simulink model "simulink_model"  (R2020b)
settings: Solver=VariableStepAuto  StartTime=0.0  StopTime=90  FixedStep=Ts  RelTol=1e-3
undefined symbols (not defined in the file): DiscIntNeverNeededParam, dist, drv, g, gbox, K, K_e_state, K_I, ms22g, Nr, Nu, Nx, sens, Ts, w_c, wheel
settings Model: Creator=giovanni  LastModifiedBy=giovanni

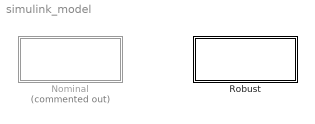
== system simulink_model ==
  Nominal : Subsystem  Commented=on
  Robust : Subsystem

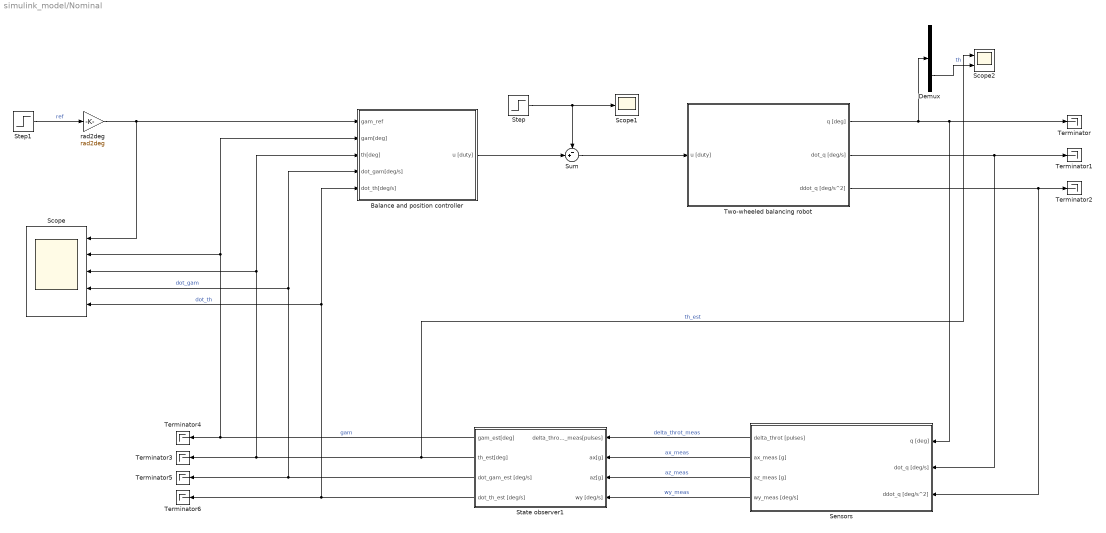
== system simulink_model/Nominal ==
  Balance and position controller : Subsystem
  Demux : Demux  Outputs=2
  Scope : Scope  NumInputPorts=5
  Scope1 : Scope
  Scope2 : Scope  NumInputPorts=2
  "Sensors " : Subsystem
  State observer1 : Subsystem
  Step : Step  Time=10  After=dist  SampleTime=Ts
  Step1 : Step  Time=0  After=step  SampleTime=0
  Sum : Sum  Inputs=-+|
  Terminator{,1..6} (7 alike) : Terminator
  Two-wheeled balancing robot : Subsystem
  rad2deg : Gain  Gain=rad2deg
  wires:
  Two-wheeled balancing robot/2(dot_q [deg/s]) -> "Sensors "/2(dot_q [deg/s]), Terminator1/1
  State observer1/3(dot_gam_est [deg/s]) -> Scope/4, Balance and position controller/4(dot_gam[deg/s]), Terminator5/1  "dot_gam"
  State observer1/4(dot_th_est [deg/s]) -> Scope/5, Balance and position controller/5(dot_th[deg/s]), Terminator6/1  "dot_th"
  Step1/1 -> rad2deg/1  "ref"
  "Sensors "/4(wy_meas [deg/s]) -> State observer1/4(wy [deg/s])  "wy_meas"
  State observer1/2(th_est[deg]) -> Scope2/1, Balance and position controller/3(th[deg]), Scope/3, Terminator3/1  "th_est"
  Two-wheeled balancing robot/3(ddot_q [deg/s^2]) -> "Sensors "/3(ddot_q [deg/s^2]), Terminator2/1
  Sum/1 -> Two-wheeled balancing robot/1(u [duty])
  "Sensors "/1(delta_throt [pulses]) -> State observer1/1(delta_throt_meas[pulses])  "delta_throt_meas"
  State observer1/1(gam_est[deg]) -> Scope/2, Balance and position controller/2(gam[deg]), Terminator4/1  "gam"
  "Sensors "/3(az_meas [g]) -> State observer1/3(az[g])  "az_meas"
  "Sensors "/2(ax_meas [g]) -> State observer1/2(ax[g])  "ax_meas"
  Two-wheeled balancing robot/1(q [deg]) -> Demux/1, "Sensors "/1(q [deg]), Terminator/1
  Balance and position controller/1(u [duty]) -> Sum/2
  Step/1 -> Scope1/1, Sum/1
  rad2deg/1 -> Scope/1, Balance and position controller/1(gam_ref)
  Demux/2 -> Scope2/2  "th"

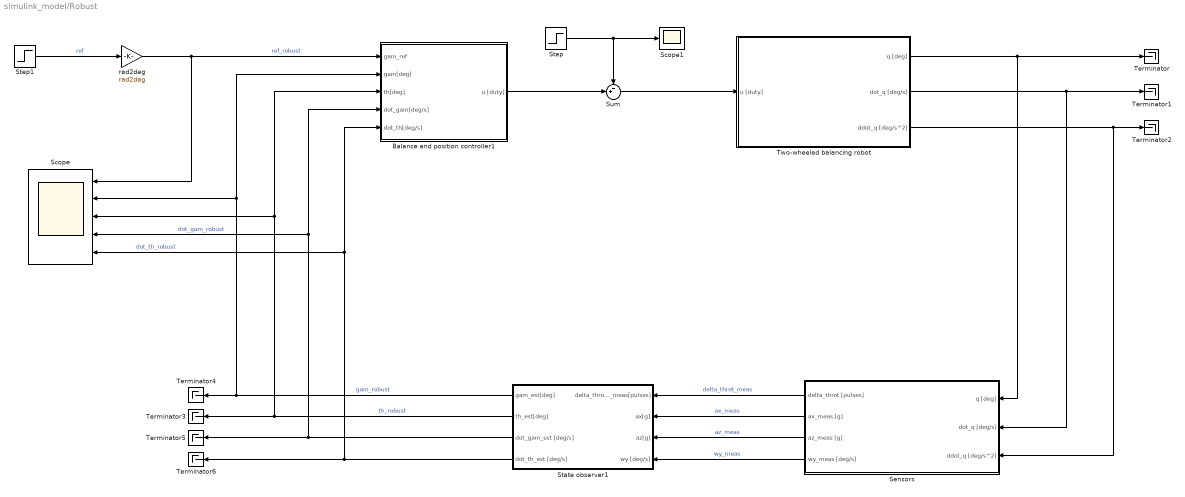
== system simulink_model/Robust ==
  Balance and position controller1 : Subsystem
  Scope : Scope  NumInputPorts=5
  Scope1 : Scope
  "Sensors " : Subsystem
  State observer1 : Subsystem
  Step : Step  Time=10  After=dist  SampleTime=Ts
  Step1 : Step  Time=0  After=step  SampleTime=0
  Sum : Sum  Inputs=-+|
  Terminator{,1..6} (7 alike) : Terminator
  Two-wheeled balancing robot : Subsystem
  rad2deg : Gain  Gain=rad2deg
  wires:
  Two-wheeled balancing robot/2(dot_q [deg/s]) -> "Sensors "/2(dot_q [deg/s]), Terminator1/1
  State observer1/3(dot_gam_est [deg/s]) -> Balance and position controller1/4(dot_gam[deg/s]), Scope/4, Terminator5/1  "dot_gam_robust"
  State observer1/4(dot_th_est [deg/s]) -> Balance and position controller1/5(dot_th[deg/s]), Scope/5, Terminator6/1  "dot_th_robust"
  Step1/1 -> rad2deg/1  "ref"
  "Sensors "/4(wy_meas [deg/s]) -> State observer1/4(wy [deg/s])  "wy_meas"
  State observer1/2(th_est[deg]) -> Balance and position controller1/3(th[deg]), Scope/3, Terminator3/1  "th_robust"
  Two-wheeled balancing robot/3(ddot_q [deg/s^2]) -> "Sensors "/3(ddot_q [deg/s^2]), Terminator2/1
  Sum/1 -> Two-wheeled balancing robot/1(u [duty])
  "Sensors "/1(delta_throt [pulses]) -> State observer1/1(delta_throt_meas[pulses])  "delta_throt_meas"
  State observer1/1(gam_est[deg]) -> Balance and position controller1/2(gam[deg]), Scope/2, Terminator4/1  "gam_robust"
  "Sensors "/3(az_meas [g]) -> State observer1/3(az[g])  "az_meas"
  "Sensors "/2(ax_meas [g]) -> State observer1/2(ax[g])  "ax_meas"
  Two-wheeled balancing robot/1(q [deg]) -> "Sensors "/1(q [deg]), Terminator/1
  Balance and position controller1/1(u [duty]) -> Sum/2
  Step/1 -> Scope1/1, Sum/1
  rad2deg/1 -> Balance and position controller1/1(gam_ref), Scope/1  "ref_robust"

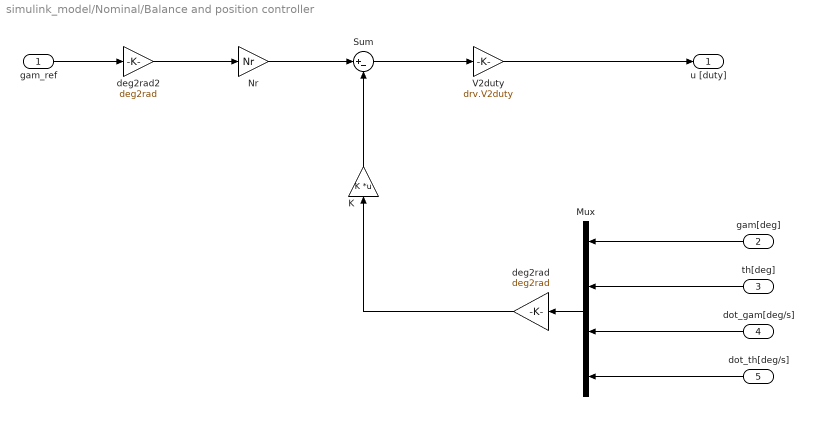
== system simulink_model/Nominal/Balance and position controller ==
  gam_ref : Inport
  gam[deg] : Inport  Port=2
  th[deg] : Inport  Port=3
  dot_gam[deg/s] : Inport  Port=4
  dot_th[deg/s] : Inport  Port=5
  K : Gain  Gain=K  Multiplication=Matrix(K*u)
  Mux : Mux
  Nr : Gain  Gain=Nr
  Sum : Sum  Inputs=|+-
  V2duty : Gain  Gain=drv.V2duty
  deg2rad : Gain  Gain=deg2rad
  deg2rad2 : Gain  Gain=deg2rad
  u [duty] : Outport
  wires:
  Nr/1 -> Sum/1
  gam_ref/1 -> deg2rad2/1
  deg2rad2/1 -> Nr/1
  Sum/1 -> V2duty/1
  V2duty/1 -> u [duty]/1
  deg2rad/1 -> K/1
  K/1 -> Sum/2
  Mux/1 -> deg2rad/1
  gam[deg]/1 -> Mux/1
  dot_th[deg/s]/1 -> Mux/4
  th[deg]/1 -> Mux/2
  dot_gam[deg/s]/1 -> Mux/3

== system simulink_model/Nominal/Sensors  ==
  q [deg] : Inport
  dot_q [deg/s] : Inport  Port=2
  ddot_q [deg/s^2] : Inport  Port=3
  Accelerometer : Subsystem
  Encoder : Subsystem
  Gyroscope : Subsystem
  delta_throt [pulses] : Outport
  ax_meas [g] : Outport  Port=2
  az_meas [g] : Outport  Port=3
  wy_meas [deg/s] : Outport  Port=4
  wires:
  ddot_q [deg/s^2]/1 -> Accelerometer/3(ddot_q [deg/s^2])
  dot_q [deg/s]/1 -> Gyroscope/1(dot_q [deg/s]), Accelerometer/2(dot_q [deg/s])
  q [deg]/1 -> Encoder/1(q [deg]), Accelerometer/1(q [deg])
  Accelerometer/1(ax [g]) -> ax_meas [g]/1
  Accelerometer/2(az [g]) -> az_meas [g]/1
  Gyroscope/1(wy [deg/s]) -> wy_meas [deg/s]/1
  Encoder/1(delta_throt [pulses]) -> delta_throt [pulses]/1

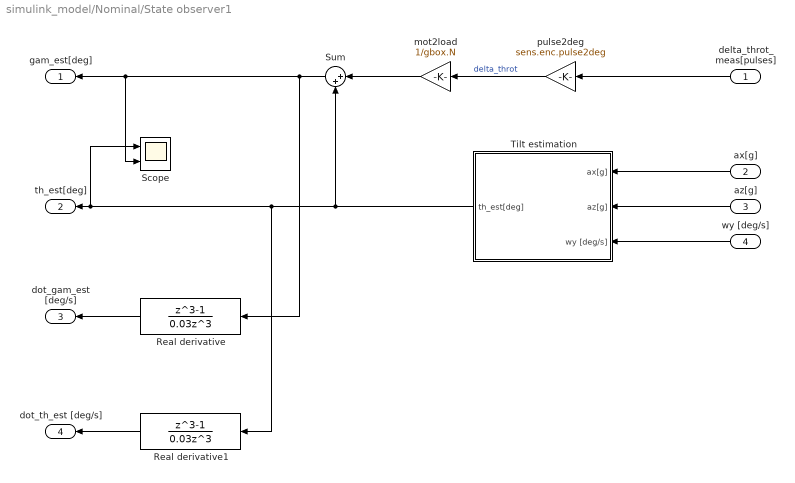
== system simulink_model/Nominal/State observer1 ==
  delta_throt_meas[pulses] : Inport
  ax[g] : Inport  Port=2
  az[g] : Inport  Port=3
  wy [deg/s] : Inport  Port=4
  Real derivative : DiscreteTransferFcn  Numerator=[1 0 0 -1]  Denominator=[0.03 0 0 0]
  Real derivative1 : DiscreteTransferFcn  Numerator=[1 0 0 -1]  Denominator=[0.03 0 0 0]
  Scope : Scope  NumInputPorts=2
  Sum : Sum  Inputs=|++
  "Tilt estimation " : Subsystem
  mot2load : Gain  Gain=1/gbox.N
  pulse2deg : Gain  Gain=sens.enc.pulse2deg
  gam_est[deg] : Outport
  th_est[deg] : Outport  Port=2
  dot_gam_est [deg/s] : Outport  Port=3
  dot_th_est [deg/s] : Outport  Port=4
  wires:
  wy [deg/s]/1 -> "Tilt estimation "/3(wy [deg/s])
  ax[g]/1 -> "Tilt estimation "/1(ax[g])
  az[g]/1 -> "Tilt estimation "/2(az[g])
  delta_throt_meas[pulses]/1 -> pulse2deg/1
  pulse2deg/1 -> mot2load/1  "delta_throt"
  mot2load/1 -> Sum/1
  "Tilt estimation "/1(th_est[deg]) -> Scope/1, th_est[deg]/1, Real derivative1/1, Sum/2
  Sum/1 -> Scope/2, gam_est[deg]/1, Real derivative/1
  Real derivative/1 -> dot_gam_est [deg/s]/1
  Real derivative1/1 -> dot_th_est [deg/s]/1

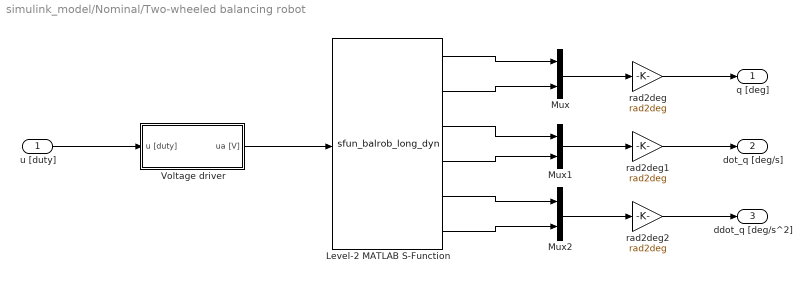
== system simulink_model/Nominal/Two-wheeled balancing robot ==
  u [duty] : Inport
  Level-2 MATLAB S-Function : M-S-Function  FunctionName=sfun_balrob_long_dyn  Parameters=x0, body, mot, gbox, wheel
  Mux : Mux  Inputs=2
  Mux1 : Mux  Inputs=2
  Mux2 : Mux  Inputs=2
  Voltage driver : Subsystem
  rad2deg : Gain  Gain=rad2deg
  rad2deg1 : Gain  Gain=rad2deg
  rad2deg2 : Gain  Gain=rad2deg
  q [deg] : Outport
  dot_q [deg/s] : Outport  Port=2
  ddot_q [deg/s^2] : Outport  Port=3
  wires:
  Level-2 MATLAB S-Function/2 -> Mux/2
  rad2deg2/1 -> ddot_q [deg/s^2]/1
  Level-2 MATLAB S-Function/1 -> Mux/1
  Mux/1 -> rad2deg/1
  rad2deg/1 -> q [deg]/1
  Level-2 MATLAB S-Function/5 -> Mux2/1
  Mux2/1 -> rad2deg2/1
  Level-2 MATLAB S-Function/4 -> Mux1/2
  Mux1/1 -> rad2deg1/1
  Level-2 MATLAB S-Function/3 -> Mux1/1
  rad2deg1/1 -> dot_q [deg/s]/1
  Level-2 MATLAB S-Function/6 -> Mux2/2
  Voltage driver/1(ua [V]) -> Level-2 MATLAB S-Function/1
  u [duty]/1 -> Voltage driver/1(u [duty])

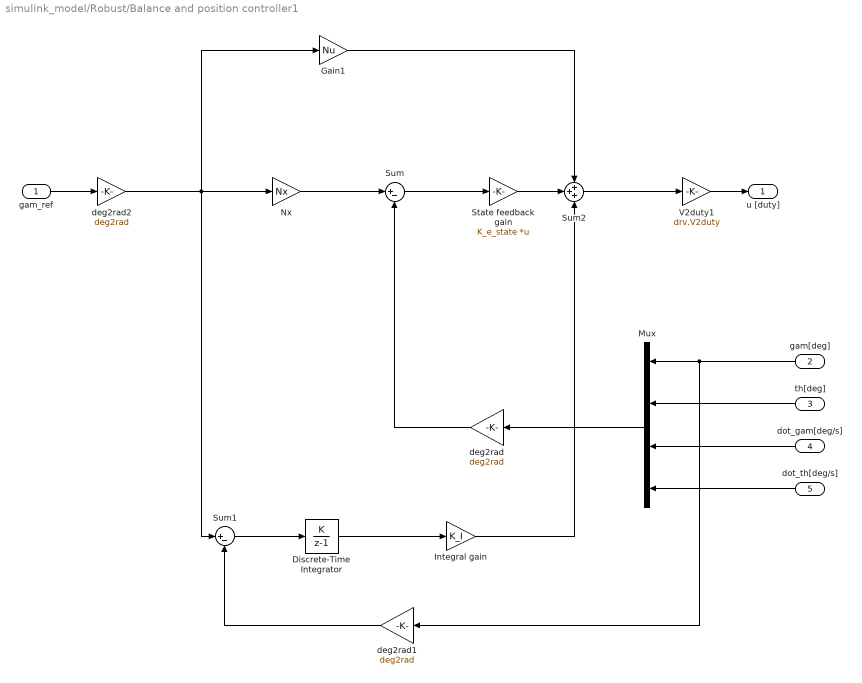
== system simulink_model/Robust/Balance and position controller1 ==
  gam_ref : Inport
  gam[deg] : Inport  Port=2
  th[deg] : Inport  Port=3
  dot_gam[deg/s] : Inport  Port=4
  dot_th[deg/s] : Inport  Port=5
  Discrete-Time Integrator : DiscreteIntegrator  IntegratorMethod=Accumulation: Forward Euler  SampleTime=-1  ICPrevOutput=DiscIntNeverNeededParam  ICPrevScaledInput=DiscIntNeverNeededParam
  Gain1 : Gain  Gain=Nu
  Integral gain : Gain  Gain=K_I
  Mux : Mux
  Nx : Gain  Gain=Nx
  State feedback gain : Gain  Gain=K_e_state  Multiplication=Matrix(K*u)
  Sum : Sum  Inputs=|+-
  Sum1 : Sum  Inputs=|+-
  Sum2 : Sum  Inputs=+++
  V2duty1 : Gain  Gain=drv.V2duty
  deg2rad : Gain  Gain=deg2rad
  deg2rad1 : Gain  Gain=deg2rad
  deg2rad2 : Gain  Gain=deg2rad
  u [duty] : Outport
  wires:
  Nx/1 -> Sum/1
  gam_ref/1 -> deg2rad2/1
  deg2rad2/1 -> Gain1/1, Sum1/1, Nx/1
  V2duty1/1 -> u [duty]/1
  deg2rad/1 -> Sum/2
  Mux/1 -> deg2rad/1
  dot_th[deg/s]/1 -> Mux/4
  th[deg]/1 -> Mux/2
  dot_gam[deg/s]/1 -> Mux/3
  gam[deg]/1 -> deg2rad1/1, Mux/1
  deg2rad1/1 -> Sum1/2
  Sum1/1 -> Discrete-Time Integrator/1
  Discrete-Time Integrator/1 -> Integral gain/1
  Sum/1 -> State feedback gain/1
  Integral gain/1 -> Sum2/3
  Gain1/1 -> Sum2/1
  State feedback gain/1 -> Sum2/2
  Sum2/1 -> V2duty1/1

== system simulink_model/Robust/Sensors  ==
  q [deg] : Inport
  dot_q [deg/s] : Inport  Port=2
  ddot_q [deg/s^2] : Inport  Port=3
  Accelerometer : Subsystem
  Encoder : Subsystem
  Gyroscope : Subsystem
  delta_throt [pulses] : Outport
  ax_meas [g] : Outport  Port=2
  az_meas [g] : Outport  Port=3
  wy_meas [deg/s] : Outport  Port=4
  wires:
  ddot_q [deg/s^2]/1 -> Accelerometer/3(ddot_q [deg/s^2])
  dot_q [deg/s]/1 -> Gyroscope/1(dot_q [deg/s]), Accelerometer/2(dot_q [deg/s])
  q [deg]/1 -> Encoder/1(q [deg]), Accelerometer/1(q [deg])
  Accelerometer/1(ax [g]) -> ax_meas [g]/1
  Accelerometer/2(az [g]) -> az_meas [g]/1
  Gyroscope/1(wy [deg/s]) -> wy_meas [deg/s]/1
  Encoder/1(delta_throt [pulses]) -> delta_throt [pulses]/1

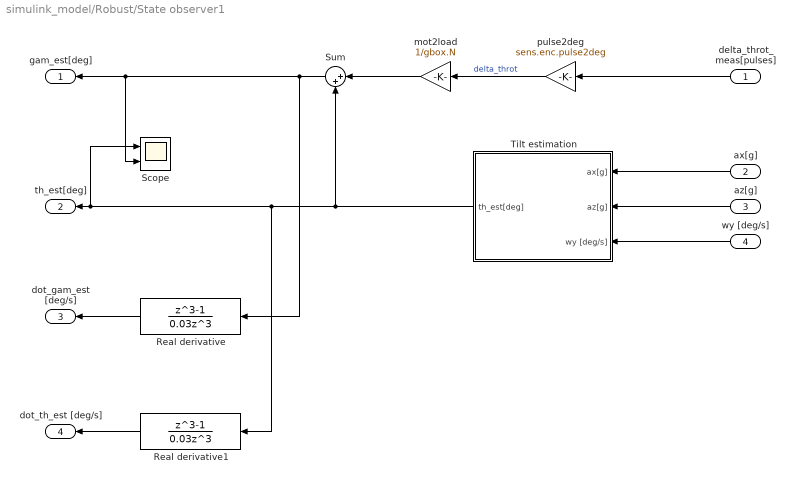
== system simulink_model/Robust/State observer1 ==
  delta_throt_meas[pulses] : Inport
  ax[g] : Inport  Port=2
  az[g] : Inport  Port=3
  wy [deg/s] : Inport  Port=4
  Real derivative : DiscreteTransferFcn  Numerator=[1 0 0 -1]  Denominator=[0.03 0 0 0]
  Real derivative1 : DiscreteTransferFcn  Numerator=[1 0 0 -1]  Denominator=[0.03 0 0 0]
  Scope : Scope  NumInputPorts=2
  Sum : Sum  Inputs=|++
  "Tilt estimation " : Subsystem
  mot2load : Gain  Gain=1/gbox.N
  pulse2deg : Gain  Gain=sens.enc.pulse2deg
  gam_est[deg] : Outport
  th_est[deg] : Outport  Port=2
  dot_gam_est [deg/s] : Outport  Port=3
  dot_th_est [deg/s] : Outport  Port=4
  wires:
  wy [deg/s]/1 -> "Tilt estimation "/3(wy [deg/s])
  ax[g]/1 -> "Tilt estimation "/1(ax[g])
  az[g]/1 -> "Tilt estimation "/2(az[g])
  delta_throt_meas[pulses]/1 -> pulse2deg/1
  pulse2deg/1 -> mot2load/1  "delta_throt"
  mot2load/1 -> Sum/1
  "Tilt estimation "/1(th_est[deg]) -> Scope/1, th_est[deg]/1, Real derivative1/1, Sum/2
  Sum/1 -> Scope/2, gam_est[deg]/1, Real derivative/1
  Real derivative/1 -> dot_gam_est [deg/s]/1
  Real derivative1/1 -> dot_th_est [deg/s]/1

== system simulink_model/Robust/Two-wheeled balancing robot ==
  u [duty] : Inport
  Level-2 MATLAB S-Function : M-S-Function  FunctionName=sfun_balrob_long_dyn  Parameters=x0, body, mot, gbox, wheel
  Mux : Mux  Inputs=2
  Mux1 : Mux  Inputs=2
  Mux2 : Mux  Inputs=2
  Voltage driver : Subsystem
  rad2deg : Gain  Gain=rad2deg
  rad2deg1 : Gain  Gain=rad2deg
  rad2deg2 : Gain  Gain=rad2deg
  q [deg] : Outport
  dot_q [deg/s] : Outport  Port=2
  ddot_q [deg/s^2] : Outport  Port=3
  wires:
  Level-2 MATLAB S-Function/2 -> Mux/2
  rad2deg2/1 -> ddot_q [deg/s^2]/1
  Level-2 MATLAB S-Function/1 -> Mux/1
  Mux/1 -> rad2deg/1
  rad2deg/1 -> q [deg]/1
  Level-2 MATLAB S-Function/5 -> Mux2/1
  Mux2/1 -> rad2deg2/1
  Level-2 MATLAB S-Function/4 -> Mux1/2
  Mux1/1 -> rad2deg1/1
  Level-2 MATLAB S-Function/3 -> Mux1/1
  rad2deg1/1 -> dot_q [deg/s]/1
  Level-2 MATLAB S-Function/6 -> Mux2/2
  Voltage driver/1(ua [V]) -> Level-2 MATLAB S-Function/1
  u [duty]/1 -> Voltage driver/1(u [duty])

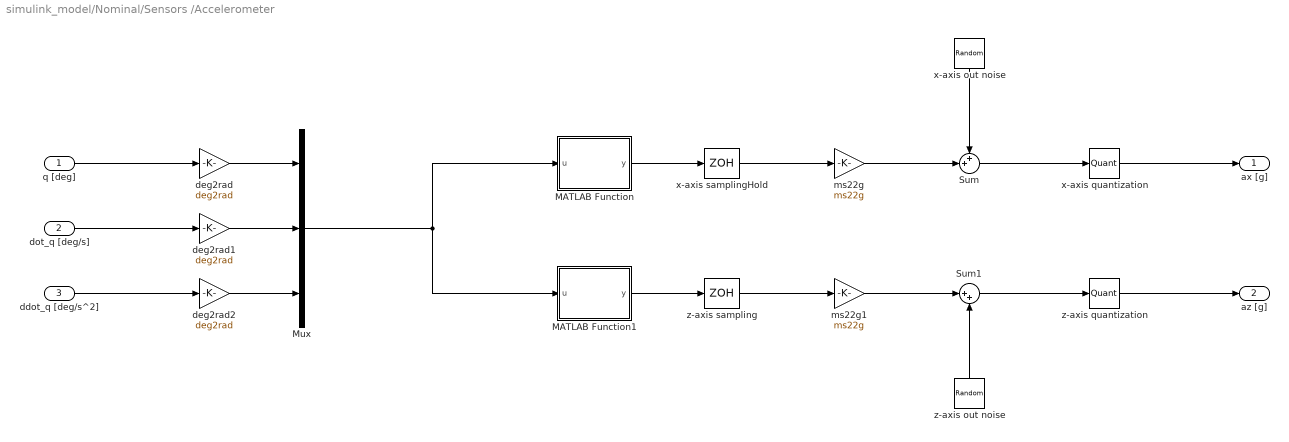
== system simulink_model/Nominal/Sensors /Accelerometer ==
  q [deg] : Inport
  dot_q [deg/s] : Inport  Port=2
  ddot_q [deg/s^2] : Inport  Port=3
  MATLAB Function : MATLAB Function  TreatAsAtomicUnit=on
  MATLAB Function1 : MATLAB Function  TreatAsAtomicUnit=on
  Mux : Mux  Inputs=3
  Sum : Sum  Inputs=++|
  Sum1 : Sum  Inputs=|++
  deg2rad : Gain  Gain=deg2rad
  deg2rad1 : Gain  Gain=deg2rad
  deg2rad2 : Gain  Gain=deg2rad
  ms22g : Gain  Gain=ms22g
  ms22g1 : Gain  Gain=ms22g
  "x-axis out noise " : RandomNumber  Variance=sens.mpu.acc.noisevar  SampleTime=Ts
  x-axis quantization : Quantizer  QuantizationInterval=sens.mpu.acc.LSB2g
  x-axis samplingHold : ZeroOrderHold  SampleTime=Ts
  "z-axis out noise " : RandomNumber  Variance=sens.mpu.acc.noisevar  SampleTime=Ts
  z-axis quantization : Quantizer  QuantizationInterval=sens.mpu.acc.LSB2g
  z-axis sampling : ZeroOrderHold  SampleTime=Ts
  ax [g] : Outport
  az [g] : Outport  Port=2
  wires:
  q [deg]/1 -> deg2rad/1
  dot_q [deg/s]/1 -> deg2rad1/1
  ddot_q [deg/s^2]/1 -> deg2rad2/1
  deg2rad/1 -> Mux/1
  deg2rad1/1 -> Mux/2
  deg2rad2/1 -> Mux/3
  Mux/1 -> MATLAB Function1/1(u), MATLAB Function/1(u)
  MATLAB Function1/1(y) -> z-axis sampling/1
  MATLAB Function/1(y) -> x-axis samplingHold/1
  x-axis samplingHold/1 -> ms22g/1
  z-axis sampling/1 -> ms22g1/1
  ms22g/1 -> Sum/2
  "x-axis out noise "/1 -> Sum/1
  ms22g1/1 -> Sum1/1
  "z-axis out noise "/1 -> Sum1/2
  Sum1/1 -> z-axis quantization/1
  Sum/1 -> x-axis quantization/1
  x-axis quantization/1 -> ax [g]/1
  z-axis quantization/1 -> az [g]/1

== system simulink_model/Nominal/Sensors /Encoder ==
  q [deg] : Inport
  Demux1 : Demux  Outputs=2
  Encoder quantization : Quantizer  QuantizationInterval=sens.enc.pulse2deg
  Encoder sampling : ZeroOrderHold  SampleTime=Ts
  Sum : Sum  Inputs=+-
  deg2pulse : Gain  Gain=sens.enc.deg2pulse
  load2mot : Gain  Gain=gbox.N
  delta_throt [pulses] : Outport
  wires:
  q [deg]/1 -> Demux1/1
  Demux1/1 -> Sum/1
  Demux1/2 -> Sum/2
  Sum/1 -> load2mot/1
  load2mot/1 -> Encoder sampling/1  "delta_throt"
  Encoder sampling/1 -> Encoder quantization/1
  Encoder quantization/1 -> deg2pulse/1
  deg2pulse/1 -> delta_throt [pulses]/1

== system simulink_model/Nominal/Sensors /Gyroscope ==
  dot_q [deg/s] : Inport
  Quantizer : Quantizer  QuantizationInterval=sens.mpu.gyro.LSB2degs
  Random Number : RandomNumber  Variance=sens.mpu.gyro.noisevar  SampleTime=Ts
  Selector : Selector  InputPortWidth=2  IndexOptions=Index vector (dialog)  Indices=[2]  OutputSizes=1
  Sum : Sum  Inputs=++|
  y-axis sampling : ZeroOrderHold  SampleTime=Ts
  wy [deg/s] : Outport
  wires:
  dot_q [deg/s]/1 -> Selector/1
  Selector/1 -> y-axis sampling/1
  y-axis sampling/1 -> Sum/2
  Sum/1 -> Quantizer/1
  Quantizer/1 -> wy [deg/s]/1
  Random Number/1 -> Sum/1

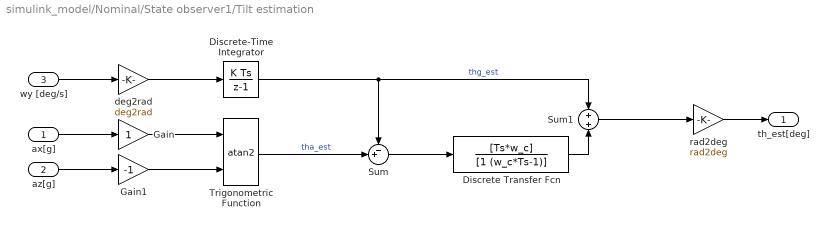
== system simulink_model/Nominal/State observer1/Tilt estimation  ==
  ax[g] : Inport
  az[g] : Inport  Port=2
  wy [deg/s] : Inport  Port=3
  Discrete Transfer Fcn : DiscreteTransferFcn  Numerator=[Ts*w_c]  Denominator=[1 (w_c*Ts-1)]  SampleTime=Ts
  Discrete-Time Integrator : DiscreteIntegrator  SampleTime=Ts  ICPrevOutput=DiscIntNeverNeededParam  ICPrevScaledInput=DiscIntNeverNeededParam
  Gain : Gain
  Gain1 : Gain  Gain=-1
  Sum : Sum  Inputs=-+|
  Sum1 : Sum  Inputs=+|+
  Trigonometric Function : Trigonometry  Operator=atan2
  deg2rad : Gain  Gain=deg2rad
  rad2deg : Gain  Gain=rad2deg
  th_est[deg] : Outport
  wires:
  wy [deg/s]/1 -> deg2rad/1
  az[g]/1 -> Gain1/1
  ax[g]/1 -> Gain/1
  deg2rad/1 -> Discrete-Time Integrator/1
  Gain/1 -> Trigonometric Function/1
  Gain1/1 -> Trigonometric Function/2
  Trigonometric Function/1 -> Sum/2  "tha_est"
  Discrete-Time Integrator/1 -> Sum1/1, Sum/1  "thg_est"
  Sum/1 -> Discrete Transfer Fcn/1
  Discrete Transfer Fcn/1 -> Sum1/2
  Sum1/1 -> rad2deg/1
  rad2deg/1 -> th_est[deg]/1

== system simulink_model/Nominal/Two-wheeled balancing robot/Voltage driver ==
  u [duty] : Inport
  Duty saturation : Saturate  UpperLimit=drv.dutymax  LowerLimit=-drv.dutymax
  Rounding Function : Rounding  Operator=fix
  Zero-Order Hold : ZeroOrderHold  SampleTime=Ts
  duty2V : Gain  Gain=drv.duty2V
  voltage saturation : Saturate  UpperLimit=drv.Vbus  LowerLimit=-drv.Vbus
  ua [V] : Outport
  wires:
  Zero-Order Hold/1 -> ua [V]/1
  duty2V/1 -> voltage saturation/1
  Rounding Function/1 -> duty2V/1
  Duty saturation/1 -> Rounding Function/1
  u [duty]/1 -> Duty saturation/1
  voltage saturation/1 -> Zero-Order Hold/1

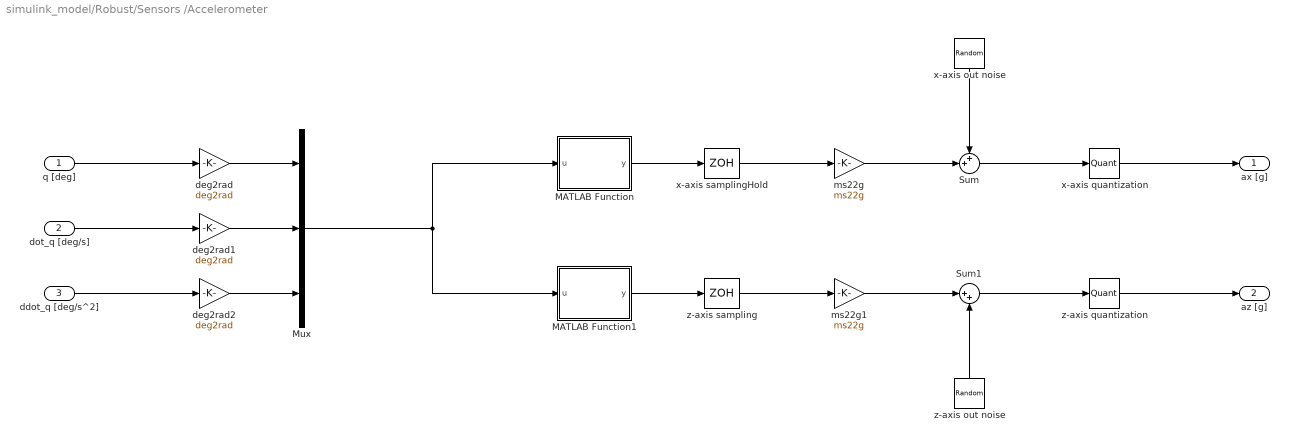
== system simulink_model/Robust/Sensors /Accelerometer ==
  q [deg] : Inport
  dot_q [deg/s] : Inport  Port=2
  ddot_q [deg/s^2] : Inport  Port=3
  MATLAB Function : MATLAB Function  TreatAsAtomicUnit=on
  MATLAB Function1 : MATLAB Function  TreatAsAtomicUnit=on
  Mux : Mux  Inputs=3
  Sum : Sum  Inputs=++|
  Sum1 : Sum  Inputs=|++
  deg2rad : Gain  Gain=deg2rad
  deg2rad1 : Gain  Gain=deg2rad
  deg2rad2 : Gain  Gain=deg2rad
  ms22g : Gain  Gain=ms22g
  ms22g1 : Gain  Gain=ms22g
  "x-axis out noise " : RandomNumber  Variance=sens.mpu.acc.noisevar  SampleTime=Ts
  x-axis quantization : Quantizer  QuantizationInterval=sens.mpu.acc.LSB2g
  x-axis samplingHold : ZeroOrderHold  SampleTime=Ts
  "z-axis out noise " : RandomNumber  Variance=sens.mpu.acc.noisevar  SampleTime=Ts
  z-axis quantization : Quantizer  QuantizationInterval=sens.mpu.acc.LSB2g
  z-axis sampling : ZeroOrderHold  SampleTime=Ts
  ax [g] : Outport
  az [g] : Outport  Port=2
  wires:
  q [deg]/1 -> deg2rad/1
  dot_q [deg/s]/1 -> deg2rad1/1
  ddot_q [deg/s^2]/1 -> deg2rad2/1
  deg2rad/1 -> Mux/1
  deg2rad1/1 -> Mux/2
  deg2rad2/1 -> Mux/3
  Mux/1 -> MATLAB Function1/1(u), MATLAB Function/1(u)
  MATLAB Function1/1(y) -> z-axis sampling/1
  MATLAB Function/1(y) -> x-axis samplingHold/1
  x-axis samplingHold/1 -> ms22g/1
  z-axis sampling/1 -> ms22g1/1
  ms22g/1 -> Sum/2
  "x-axis out noise "/1 -> Sum/1
  ms22g1/1 -> Sum1/1
  "z-axis out noise "/1 -> Sum1/2
  Sum1/1 -> z-axis quantization/1
  Sum/1 -> x-axis quantization/1
  x-axis quantization/1 -> ax [g]/1
  z-axis quantization/1 -> az [g]/1

== system simulink_model/Robust/Sensors /Encoder ==
  q [deg] : Inport
  Demux1 : Demux  Outputs=2
  Encoder quantization : Quantizer  QuantizationInterval=sens.enc.pulse2deg
  Encoder sampling : ZeroOrderHold  SampleTime=Ts
  Sum : Sum  Inputs=+-
  deg2pulse : Gain  Gain=sens.enc.deg2pulse
  load2mot : Gain  Gain=gbox.N
  delta_throt [pulses] : Outport
  wires:
  q [deg]/1 -> Demux1/1
  Demux1/1 -> Sum/1
  Demux1/2 -> Sum/2
  Sum/1 -> load2mot/1
  load2mot/1 -> Encoder sampling/1  "delta_throt"
  Encoder sampling/1 -> Encoder quantization/1
  Encoder quantization/1 -> deg2pulse/1
  deg2pulse/1 -> delta_throt [pulses]/1

== system simulink_model/Robust/Sensors /Gyroscope ==
  dot_q [deg/s] : Inport
  Quantizer : Quantizer  QuantizationInterval=sens.mpu.gyro.LSB2degs
  Random Number : RandomNumber  Variance=sens.mpu.gyro.noisevar  SampleTime=Ts
  Selector : Selector  InputPortWidth=2  IndexOptions=Index vector (dialog)  Indices=[2]  OutputSizes=1
  Sum : Sum  Inputs=++|
  y-axis sampling : ZeroOrderHold  SampleTime=Ts
  wy [deg/s] : Outport
  wires:
  dot_q [deg/s]/1 -> Selector/1
  Selector/1 -> y-axis sampling/1
  y-axis sampling/1 -> Sum/2
  Sum/1 -> Quantizer/1
  Quantizer/1 -> wy [deg/s]/1
  Random Number/1 -> Sum/1

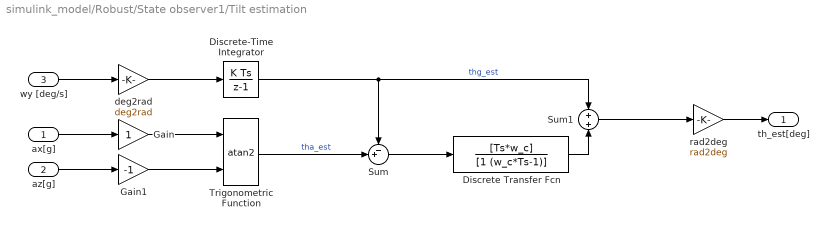
== system simulink_model/Robust/State observer1/Tilt estimation  ==
  ax[g] : Inport
  az[g] : Inport  Port=2
  wy [deg/s] : Inport  Port=3
  Discrete Transfer Fcn : DiscreteTransferFcn  Numerator=[Ts*w_c]  Denominator=[1 (w_c*Ts-1)]  SampleTime=Ts
  Discrete-Time Integrator : DiscreteIntegrator  SampleTime=Ts  ICPrevOutput=DiscIntNeverNeededParam  ICPrevScaledInput=DiscIntNeverNeededParam
  Gain : Gain
  Gain1 : Gain  Gain=-1
  Sum : Sum  Inputs=-+|
  Sum1 : Sum  Inputs=+|+
  Trigonometric Function : Trigonometry  Operator=atan2
  deg2rad : Gain  Gain=deg2rad
  rad2deg : Gain  Gain=rad2deg
  th_est[deg] : Outport
  wires:
  wy [deg/s]/1 -> deg2rad/1
  az[g]/1 -> Gain1/1
  ax[g]/1 -> Gain/1
  deg2rad/1 -> Discrete-Time Integrator/1
  Gain/1 -> Trigonometric Function/1
  Gain1/1 -> Trigonometric Function/2
  Trigonometric Function/1 -> Sum/2  "tha_est"
  Discrete-Time Integrator/1 -> Sum1/1, Sum/1  "thg_est"
  Sum/1 -> Discrete Transfer Fcn/1
  Discrete Transfer Fcn/1 -> Sum1/2
  Sum1/1 -> rad2deg/1
  rad2deg/1 -> th_est[deg]/1

== system simulink_model/Robust/Two-wheeled balancing robot/Voltage driver ==
  u [duty] : Inport
  Duty saturation : Saturate  UpperLimit=drv.dutymax  LowerLimit=-drv.dutymax
  Rounding Function : Rounding  Operator=fix
  Zero-Order Hold : ZeroOrderHold  SampleTime=Ts
  duty2V : Gain  Gain=drv.duty2V
  voltage saturation : Saturate  UpperLimit=drv.Vbus  LowerLimit=-drv.Vbus
  ua [V] : Outport
  wires:
  Zero-Order Hold/1 -> ua [V]/1
  duty2V/1 -> voltage saturation/1
  Rounding Function/1 -> duty2V/1
  Duty saturation/1 -> Rounding Function/1
  u [duty]/1 -> Duty saturation/1
  voltage saturation/1 -> Zero-Order Hold/1

== matlab function simulink_model/Robust/Sensors /Accelerometer/MATLAB Function ==
  data: u input; y output; wheel parameter; sens parameter; g parameter
function y = acc_out_x(u, wheel, sens, g)

y = wheel.r*u(5)*cos(u(2)) + sens.mpu.zb*u(6) + g*sin(u(2));

== matlab function simulink_model/Robust/Sensors /Accelerometer/MATLAB Function1 ==
  data: u input; y output; wheel parameter; sens parameter; g parameter
function y = acc_out_z(u, wheel, sens, g)

y = wheel.r*u(5)*sin(u(2)) - sens.mpu.zb*u(4)^2 - g*cos(u(2));

== matlab function simulink_model/Nominal/Sensors /Accelerometer/MATLAB Function ==
  data: u input; y output; wheel parameter; sens parameter; g parameter
function y = acc_out_x(u, wheel, sens, g)

y = wheel.r*u(5)*cos(u(2)) + sens.mpu.zb*u(6) + g*sin(u(2));

== matlab function simulink_model/Nominal/Sensors /Accelerometer/MATLAB Function1 ==
  data: u input; y output; wheel parameter; sens parameter; g parameter
function y = acc_out_z(u, wheel, sens, g)

y = wheel.r*u(5)*sin(u(2)) - sens.mpu.zb*u(4)^2 - g*cos(u(2));
